simulink model "TestMidiInput"  (R2018b)
settings: Solver=VariableStepAuto  StartTime=0.0  StopTime=inf  RelTol=1e-3
settings Model: Creator=asus  LastModifiedBy=asus

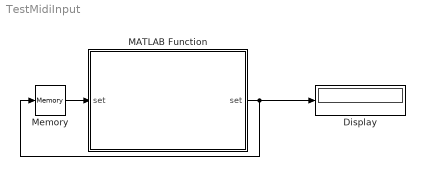
== system TestMidiInput ==
  Display : Display
  MATLAB Function : MATLAB Function  TreatAsAtomicUnit=on
  Memory : Memory
  wires:
  MATLAB Function/1(set) -> Memory/1, Display/1
  Memory/1 -> MATLAB Function/1("set ")

== matlab function TestMidiInput/MATLAB Function ==
  data: set input; set output
function set = parseInput(set)
% code taken and modified from matlab's given simple synth

midiDeviceName = 'Yamaha S08-1';
midiInput = mididevice(midiDeviceName);

    while true
        msgs = midireceive(midiInput);
        for i = 1:numel(msgs)
            msg = msgs(i);
            if isNoteOn(msg)             
                set = union(set, msg.Note);
            elseif isNoteOff(msg)
                set = setdiff(set, msg.Note);
            end
        end
    end
end

function yes = isNoteOn(msg)
    yes = msg.Type == midimsgtype.NoteOn ...
        && msg.Velocity > 0;
end

function yes = isNoteOff(msg)
    yes = msg.Type == midimsgtype.NoteOff ...
        || (msg.Type == midimsgtype.NoteOn && msg.Velocity == 0);
end
